simulink model "Transmitter"  (R2021b)
settings: Solver=VariableStepAuto  StartTime=0.0  StopTime=10.0  RelTol=1e-3
undefined symbols (not defined in the file or in its folder): Length, Rate
settings Model: Creator=ahmad  LastModifiedBy=ahmad

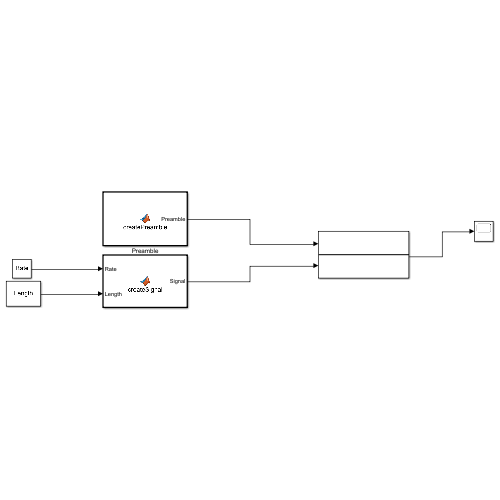
[thumbnail: Simulink's stored preview of the top-level diagram]
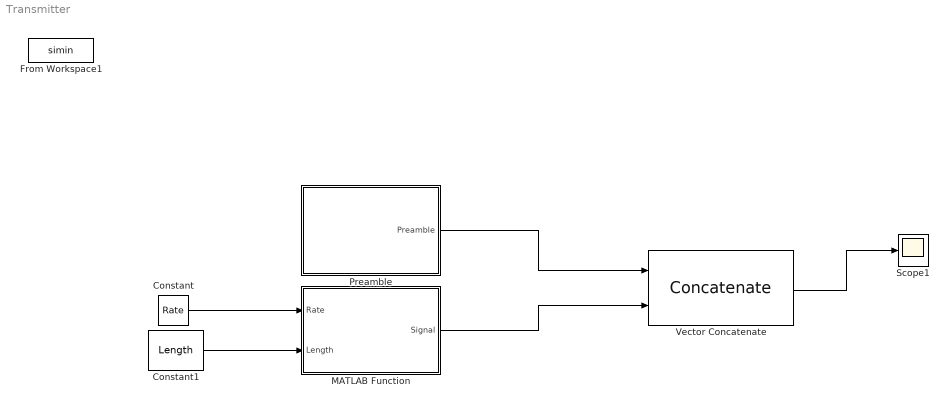
== system Transmitter ==
  Constant : Constant  Value=Rate
  Constant1 : Constant  Value=Length
  MATLAB Function : MATLAB Function  TreatAsAtomicUnit=on
  Preamble : MATLAB Function  TreatAsAtomicUnit=on
  Scope1 : Scope
  Vector Concatenate : Concatenate
  From Workspace1 : FromWorkspace  IOType=siggen  VariableName=simin  ZeroCross=off
  wires:
  Constant/1 -> MATLAB Function/1(Rate)
  Constant1/1 -> MATLAB Function/2(Length)
  Preamble/1(Preamble) -> Vector Concatenate/1
  MATLAB Function/1(Signal) -> Vector Concatenate/2
  Vector Concatenate/1 -> Scope1/1

== matlab function Transmitter/Preamble ==
  data: Preamble output
function Preamble = createPreamble()
    window = [0.5; ones(159,1); 0.5];
    ShortSymbol = sqrt(13/6) * [0,0,0,0,0,0,0, 0, 1+1j, 0, 0, 0, -1-1j, 0, 0, 0, 1+1j, 0, 0, 0, -1-1j, 0, 0, 0, -1-1j, 0, 0, 0, 1+1j, 0, 0, 0, 0,...
                    0, 0, 0, -1-1j, 0, 0, 0, -1-1j, 0, 0, 0, 1+1j, 0, 0, 0, 1+1j, 0, 0, 0, 1+1j, 0, 0, 0, 1+1j, 0,0,0,0,0,0,0].';

    ShortPreamble = ofdmmod(ShortSymbol(ShortSymbol~=0),64,0, ...
        find(ShortSymbol == 0));
    ShortPreamble = [ShortPreamble;ShortPreamble;ShortPreamble(1:(160-128+1))];
    
    ShortPreamble = ShortPreamble .* window;
    
    LongSymbol = [1, 1, -1, -1, 1, 1, -1, 1, -1, 1, 1, 1, 1, 1, 1, -1, -1, 1,...
                  1, -1, 1, -1, 1, 1, 1, 1, 1, -1, -1, 1, 1, -1, 1, -1, 1,...
                  -1, -1, -1, -1, -1, 1, 1, -1, -1, 1, -1, 1, -1, 1, 1, 1, 1].';
    LongPreamble = [ofdmmod(LongSymbol, 64, 32,  [1:6 33 64-4:64].');ofdmmod(LongSymbol, 64, 0,  [1:6 33 64-4:64].')];
    LongPreamble = window .* [LongPreamble;LongPreamble(33)];
    
    Preamble = [ShortPreamble(1:end-1); ShortPreamble(end)+LongPreamble(1); LongPreamble(2:end)];
end

== matlab function Transmitter/MATLAB Function ==
  data: Rate input; Signal output; Length input
function Signal = createSignal(Rate, Length)
    Tail = uint8(zeros(6,1));
    window = [0.5; ones(78,1); 0.5];
    RateTable = containers.Map({3, 4.5, 6, 9, 12, 18, 24, 27},...
               {uint8([1 1 0 1]), uint8([1 1 1 1]), uint8([0 1 0 1]),...
               uint8([0 1 1 1]), uint8([1 0 0 1]), uint8([1 0 1 1]),...
               uint8([0 0 0 1]), uint8([0 0 1 1])});
    RateBits = RateTable(Rate).';
    LengthBits = uint8(flipud(int2bit(Length,12)));
    ParityBit = uint8(mod(sum([RateBits;0;LengthBits]),2));
    SignalBits = [RateBits;0;LengthBits;ParityBit;Tail];
    SignalBits = convenc(SignalBits,poly2trellis(7,[133 171]));
    SignalBits = Interleaver(SignalBits,48);
    Signal = pskmod(SignalBits,2,pi);
    Signal = insertPilots(Signal,0);
    Signal = window .* ofdmmod(Signal,64,16,[1:6 33 60:64].');
end
